simulink model "CtrlStrct_VNT_Level1_TW"  (R2018a)
settings: Solver=FixedStepAuto  StartTime=0.0  StopTime=10.0  FixedStep=0.001  RelTol=1e-3  EnableMultiTasking=on
PreLoadFcn:
  | CtrlStrct_SmplCAN_BusInfo
libraries: canmsglib x55, simulink x1
(part 3 of 3)

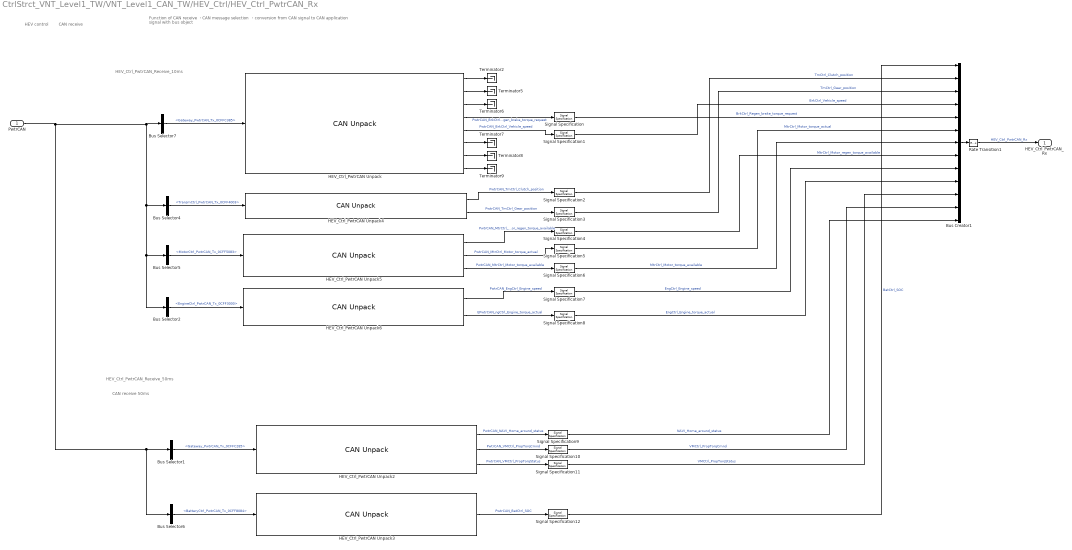
== system CtrlStrct_VNT_Level1_TW/VNT_Level1_CAN_TW/HEV_Ctrl/HEV_Ctrl_PwtrCAN_Rx ==
  note: HEV_Ctrl_PwtrCAN_Receive_50ms
  note: HEV_Ctrl_PwtrCAN_Receive_10ms
  note: CAN receive
  note: HEV control
  note: Function of CAN receive
      | ・CAN message selection
      | ・conversion from CAN signal to CAN application signal with bus object
  note: CAN receive 50ms
  PwtrCAN : Inport
  Bus Creator1 : BusCreator  Inputs=13  OutDataTypeStr=Bus: HEV_Ctrl_PwtrCAN_Rx_Bus
  Bus Selector1 : BusSelector  OutputSignals=Gateway_PwtrCAN_Tx_0CFFC285
  Bus Selector2 : BusSelector  OutputSignals=EngineCtrl_PwtrCAN_Tx_0CFF3000
  Bus Selector4 : BusSelector  OutputSignals=TransmCtrl_PwtrCAN_Tx_0CFF4003
  Bus Selector5 : BusSelector  OutputSignals=MotorCtrl_PwtrCAN_Tx_0CFF5083
  Bus Selector6 : BusSelector  OutputSignals=BatteryCtrl_PwtrCAN_Tx_0CFF8084
  Bus Selector7 : BusSelector  OutputSignals=Gateway_PwtrCAN_Tx_0CFFC385
  HEV_Ctrl_PwtrCAN Unpack : canmsglib/CAN Unpack  CANdbFile=HEV_CANDB.dbc  MsgList=Gateway_PwtrCAN_Tx_2  MsgName=Gateway_PwtrCAN_Tx_2  MsgIDType=Extended (29-bit identifier)  MsgIdentifier=218088325  MsgLength=8  SignalInfo=BdyCtrl_Door_open_flag_G$60$1$1$2$1$0$1$0$0$1$#BdyCtrl_Engine_hood_open_flg_G$59$1$1$2$1$0$1$0$0$1$#BdyCtrl_Idlestop_cancel_G$58$1$1$2$1$0$1$0$0$1$#BrkCtrl_Regen_brake_torque_re_G$16$16$1$1$1$0$1.000000e-02$0$-300$300$#BrkCtrl_Vehicle_speed_G$0$16$1$2$1$0$1.000000e-01$0$0$180$#HVAC_Ctrl_Idlestop_cancel_G$57$1$1$2$1$0$1$0$0$1$#HVAC_Ctrl_Idlestop_enbl_G$56$1$1$2$1$0$1$0$0$1$#StrgCtrl_Steer_angle_G$32$16$1$1$1$0$3.125000e-02$0$-720$720$#  NSignals=8  IDPort=off  TimestampPort=off  ErrorPort=off  RemotePort=off  LengthPort=off  StatusPort=off  StartBits=str2num('[int32(60);int32(59);int32(58);int32(16);int32(0);int32(57);int32(56);int32(32)]')  SignalSizes=str2num('[int32(1);int32(1);int32(1);int32(16);int32(16);int32(1);int32(1);int32(16)]')  ByteOrders=str2num('[int32(1);int32(1);int32(1);int32(1);int32(1);int32(1);int32(1);int32(1)]')  DataTypes=str2num('[int32(2);int32(2);int32(2);int32(1);int32(2);int32(2);int32(2);int32(1)]')  MultiplexTypes=str2num('[int32(1);int32(1);int32(1);int32(1);int32(1);int32(1);int32(1);int32(1)]')  MultiplexValues=str2num('[double(0);double(0);double(0);double(0);double(0);double(0);double(0);double(0)]')  Factors=str2num('[double(1);double(1);double(1);double(1.000000e-02);double(1.000000e-01);double(1);double(1);double(3.125000e-02)]')  Offsets=str2num('[double(0);double(0);double(0);double(0);double(0);double(0);double(0);double(0)]')  Minimums=str2num('[double(0);double(0);double(0);double(-300);double(0);double(0);double(0);double(-720)]')  Maximums=str2num('[double(1);double(1);double(1);double(300);double(180);double(1);double(1);double(720)]')  ApplyMinMax=off
      settings: AttributesFormatString=<CANdbFile = %<CANdbFile>>  SourceProductName=Simulink Real-Time  SourceProductBaseCode=XP  DataFormat=CANdb specified signals
  HEV_Ctrl_PwtrCAN Unpack2 : canmsglib/CAN Unpack  CANdbFile=HEV_CANDB.dbc  MsgList=Gateway_PwtrCAN_Tx_1  MsgName=Gateway_PwtrCAN_Tx_1  MsgIDType=Extended (29-bit identifier)  MsgIdentifier=218088069  MsgLength=8  SignalInfo=NAVI_Home_around_status_G$0$16$1$2$1$0$1$0$0$65535$#VMCtrl_PropTorqCmnd_G$24$16$1$1$1$0$1.000000e-02$0$-300$300$#VMCtrl_PropTorqStatus_G$16$8$1$2$1$0$1$0$0$7$#  NSignals=3  IDPort=off  TimestampPort=off  ErrorPort=off  RemotePort=off  LengthPort=off  StatusPort=off  StartBits=str2num('[int32(0);int32(24);int32(16)]')  SignalSizes=str2num('[int32(16);int32(16);int32(8)]')  ByteOrders=str2num('[int32(1);int32(1);int32(1)]')  DataTypes=str2num('[int32(2);int32(1);int32(2)]')  MultiplexTypes=str2num('[int32(1);int32(1);int32(1)]')  MultiplexValues=str2num('[double(0);double(0);double(0)]')  Factors=str2num('[double(1);double(1.000000e-02);double(1)]')  Offsets=str2num('[double(0);double(0);double(0)]')  Minimums=str2num('[double(0);double(-300);double(0)]')  Maximums=str2num('[double(65535);double(300);double(7)]')  ApplyMinMax=off
      settings: AttributesFormatString=<CANdbFile = %<CANdbFile>>  SourceProductName=Simulink Real-Time  SourceProductBaseCode=XP  DataFormat=CANdb specified signals
  HEV_Ctrl_PwtrCAN Unpack3 : canmsglib/CAN Unpack  CANdbFile=HEV_CANDB.dbc  MsgList=BatteryCtrl_PwtrCAN_Tx  MsgName=BatteryCtrl_PwtrCAN_Tx  MsgIDType=Extended (29-bit identifier)  MsgIdentifier=218071172  MsgLength=8  SignalInfo=BatCtrl_SOC$0$16$1$2$1$0$3.906250e-03$0$0$100$#  NSignals=1  IDPort=off  TimestampPort=off  ErrorPort=off  RemotePort=off  LengthPort=off  StatusPort=off  StartBits=str2num('[int32(0)]')  SignalSizes=str2num('[int32(16)]')  ByteOrders=str2num('[int32(1)]')  DataTypes=str2num('[int32(2)]')  MultiplexTypes=str2num('[int32(1)]')  MultiplexValues=str2num('[double(0)]')  Factors=str2num('[double(3.906250e-03)]')  Offsets=str2num('[double(0)]')  Minimums=str2num('[double(0)]')  Maximums=str2num('[double(100)]')  ApplyMinMax=off
      settings: AttributesFormatString=<CANdbFile = %<CANdbFile>>  SourceProductName=Simulink Real-Time  SourceProductBaseCode=XP  DataFormat=CANdb specified signals
  HEV_Ctrl_PwtrCAN Unpack4 : canmsglib/CAN Unpack  CANdbFile=HEV_CANDB.dbc  MsgList=TransmCtrl_PwtrCAN_Tx  MsgName=TransmCtrl_PwtrCAN_Tx  MsgIDType=Extended (29-bit identifier)  MsgIdentifier=218054659  MsgLength=8  SignalInfo=TmCtrl_Clutch_position$0$8$1$2$1$0$1.000000e-02$0$0$1$#TmCtrl_Gear_position$8$8$1$2$1$0$1$0$0$5$#  NSignals=2  IDPort=off  TimestampPort=off  ErrorPort=off  RemotePort=off  LengthPort=off  StatusPort=off  StartBits=str2num('[int32(0);int32(8)]')  SignalSizes=str2num('[int32(8);int32(8)]')  ByteOrders=str2num('[int32(1);int32(1)]')  DataTypes=str2num('[int32(2);int32(2)]')  MultiplexTypes=str2num('[int32(1);int32(1)]')  MultiplexValues=str2num('[double(0);double(0)]')  Factors=str2num('[double(1.000000e-02);double(1)]')  Offsets=str2num('[double(0);double(0)]')  Minimums=str2num('[double(0);double(0)]')  Maximums=str2num('[double(1);double(5)]')  ApplyMinMax=off
      settings: AttributesFormatString=<CANdbFile = %<CANdbFile>>  SourceProductName=Simulink Real-Time  SourceProductBaseCode=XP  DataFormat=CANdb specified signals
  HEV_Ctrl_PwtrCAN Unpack5 : canmsglib/CAN Unpack  CANdbFile=HEV_CANDB.dbc  MsgList=MotorCtrl_PwtrCAN_Tx  MsgName=MotorCtrl_PwtrCAN_Tx  MsgIDType=Extended (29-bit identifier)  MsgIdentifier=218058883  MsgLength=8  SignalInfo=MtrCtrl_Motor_regen_torque_avail$32$16$1$1$1$0$1.000000e-02$0$-300$300$#MtrCtrl_Motor_torque_actual$0$16$1$1$1$0$1.000000e-02$0$-300$300$#MtrCtrl_Motor_torque_available$16$16$1$1$1$0$1.000000e-02$0$-300$300$#  NSignals=3  IDPort=off  TimestampPort=off  ErrorPort=off  RemotePort=off  LengthPort=off  StatusPort=off  StartBits=str2num('[int32(32);int32(0);int32(16)]')  SignalSizes=str2num('[int32(16);int32(16);int32(16)]')  ByteOrders=str2num('[int32(1);int32(1);int32(1)]')  DataTypes=str2num('[int32(1);int32(1);int32(1)]')  MultiplexTypes=str2num('[int32(1);int32(1);int32(1)]')  MultiplexValues=str2num('[double(0);double(0);double(0)]')  Factors=str2num('[double(1.000000e-02);double(1.000000e-02);double(1.000000e-02)]')  Offsets=str2num('[double(0);double(0);double(0)]')  Minimums=str2num('[double(-300);double(-300);double(-300)]')  Maximums=str2num('[double(300);double(300);double(300)]')  ApplyMinMax=off
      settings: AttributesFormatString=<CANdbFile = %<CANdbFile>>  SourceProductName=Simulink Real-Time  SourceProductBaseCode=XP  DataFormat=CANdb specified signals
  HEV_Ctrl_PwtrCAN Unpack6 : canmsglib/CAN Unpack  CANdbFile=HEV_CANDB.dbc  MsgList=EngineCtrl_PwtrCAN_Tx  MsgName=EngineCtrl_PwtrCAN_Tx  MsgIDType=Extended (29-bit identifier)  MsgIdentifier=218050560  MsgLength=8  SignalInfo=EngCtrl_Engine_speed$0$16$1$2$1$0$1.250000e-01$0$0$8192$#EngCtrl_Engine_torque_actual$16$16$1$1$1$0$1.562500e-02$0$-300$300$#  NSignals=2  IDPort=off  TimestampPort=off  ErrorPort=off  RemotePort=off  LengthPort=off  StatusPort=off  StartBits=str2num('[int32(0);int32(16)]')  SignalSizes=str2num('[int32(16);int32(16)]')  ByteOrders=str2num('[int32(1);int32(1)]')  DataTypes=str2num('[int32(2);int32(1)]')  MultiplexTypes=str2num('[int32(1);int32(1)]')  MultiplexValues=str2num('[double(0);double(0)]')  Factors=str2num('[double(1.250000e-01);double(1.562500e-02)]')  Offsets=str2num('[double(0);double(0)]')  Minimums=str2num('[double(0);double(-300)]')  Maximums=str2num('[double(8192);double(300)]')  ApplyMinMax=off
      settings: AttributesFormatString=<CANdbFile = %<CANdbFile>>  SourceProductName=Simulink Real-Time  SourceProductBaseCode=XP  DataFormat=CANdb specified signals
  Rate Transition1 : RateTransition  Deterministic=off
      settings: AttributesFormatString=<Deterministic=%<Deterministic>>
  Signal Specification{,1..12} (13 alike) : SignalSpecification
  Terminator{2,5..9} (6 alike) : Terminator
  HEV_Ctrl_PwtrCAN_Rx : Outport
  wires:
  Rate Transition1/1 -> HEV_Ctrl_PwtrCAN_Rx/1  "HEV_Ctrl_PwtrCAN_Rx"
  Bus Creator1/1 -> Rate Transition1/1
  Signal Specification8/1 -> Bus Creator1/10  "EngCtrl_Engine_torque_actual"
  HEV_Ctrl_PwtrCAN Unpack/3 -> Terminator6/1
  HEV_Ctrl_PwtrCAN Unpack/6 -> Terminator7/1
  Signal Specification7/1 -> Bus Creator1/9  "EngCtrl_Engine_speed"
  HEV_Ctrl_PwtrCAN Unpack/1 -> Terminator2/1
  HEV_Ctrl_PwtrCAN Unpack/2 -> Terminator5/1
  HEV_Ctrl_PwtrCAN Unpack5/1 -> Signal Specification4/1  "PwtrCAN_MtrCtrl_Motor_regen_torque_available"
  Signal Specification6/1 -> Bus Creator1/7  "MtrCtrl_Motor_torque_available"
  HEV_Ctrl_PwtrCAN Unpack/5 -> Signal Specification1/1  "PwtrCAN_BrkCtrl_Vehicle_speed"
  HEV_Ctrl_PwtrCAN Unpack/4 -> Signal Specification/1  "PwtrCAN_BrkCtrl_Regen_brake_torque_request"
  HEV_Ctrl_PwtrCAN Unpack6/2 -> Signal Specification8/1  "EPwtrCAN_ngCtrl_Engine_torque_actual"
  Signal Specification2/1 -> Bus Creator1/2  "TmCtrl_Clutch_position"
  Signal Specification4/1 -> Bus Creator1/8  "MtrCtrl_Motor_regen_torque_available"
  HEV_Ctrl_PwtrCAN Unpack/8 -> Terminator9/1
  HEV_Ctrl_PwtrCAN Unpack5/2 -> Signal Specification5/1  "PwtrCAN_MtrCtrl_Motor_torque_actual"
  Signal Specification3/1 -> Bus Creator1/3  "TmCtrl_Gear_position"
  HEV_Ctrl_PwtrCAN Unpack4/1 -> Signal Specification2/1  "PwtrCAN_TmCtrl_Clutch_position"
  HEV_Ctrl_PwtrCAN Unpack6/1 -> Signal Specification7/1  "PwtrCAN_EngCtrl_Engine_speed"
  Signal Specification1/1 -> Bus Creator1/4  "BrkCtrl_Vehicle_speed"
  HEV_Ctrl_PwtrCAN Unpack4/2 -> Signal Specification3/1  "PwtrCAN_TmCtrl_Gear_position"
  HEV_Ctrl_PwtrCAN Unpack5/3 -> Signal Specification6/1  "PwtrCAN_MtrCtrl_Motor_torque_available"
  Signal Specification/1 -> Bus Creator1/5  "BrkCtrl_Regen_brake_torque_request"
  HEV_Ctrl_PwtrCAN Unpack/7 -> Terminator8/1
  Signal Specification5/1 -> Bus Creator1/6  "MtrCtrl_Motor_torque_actual"
  Bus Selector7/1 -> HEV_Ctrl_PwtrCAN Unpack/1  "<Gateway_PwtrCAN_Tx_0CFFC385>"
  Bus Selector5/1 -> HEV_Ctrl_PwtrCAN Unpack5/1  "<MotorCtrl_PwtrCAN_Tx_0CFF5083>"
  Bus Selector4/1 -> HEV_Ctrl_PwtrCAN Unpack4/1  "<TransmCtrl_PwtrCAN_Tx_0CFF4003>"
  Bus Selector2/1 -> HEV_Ctrl_PwtrCAN Unpack6/1  "<EngineCtrl_PwtrCAN_Tx_0CFF3000>"
  Signal Specification11/1 -> Bus Creator1/11  "VMCtrl_PropTorqStatus"
  Signal Specification12/1 -> Bus Creator1/1  "BatCtrl_SOC"
  HEV_Ctrl_PwtrCAN Unpack3/1 -> Signal Specification12/1  "PwtrCAN_BatCtrl_SOC"
  Signal Specification9/1 -> Bus Creator1/13  "NAVI_Home_around_status"
  Signal Specification10/1 -> Bus Creator1/12  "VMCtrl_PropTorqCmnd"
  HEV_Ctrl_PwtrCAN Unpack2/2 -> Signal Specification10/1  "PwtrCAN_VMCtrl_PropTorqCmnd"
  HEV_Ctrl_PwtrCAN Unpack2/3 -> Signal Specification11/1  "PwtrCAN_VMCtrl_PropTorqStatus"
  HEV_Ctrl_PwtrCAN Unpack2/1 -> Signal Specification9/1  "PwtrCAN_NAVI_Home_around_status"
  Bus Selector1/1 -> HEV_Ctrl_PwtrCAN Unpack2/1  "<Gateway_PwtrCAN_Tx_0CFFC285>"
  PwtrCAN/1 -> Bus Selector7/1, Bus Selector5/1, Bus Selector2/1, Bus Selector4/1, Bus Selector6/1, Bus Selector1/1
  Bus Selector6/1 -> HEV_Ctrl_PwtrCAN Unpack3/1  "<BatteryCtrl_PwtrCAN_Tx_0CFF8084>"

== system CtrlStrct_VNT_Level1_TW/VNT_Level1_CAN_TW/HVAC_Ctrl/HVAC_Ctrl_VehCAN Tx ==
  note: CAN transmit
  note: Function of CAN transmit
      | ・conversion fromCAN application signal to signal of CAN message
  note: HVAC Control
  HVAC_Ctrl_VehCAN_Tx_Apli : Inport
  Bus Creator1 : BusCreator  Inputs=1
  Bus Selector2 : BusSelector  OutputSignals=HVAC_Ctrl_Idlestop_cancel,HVAC_Ctrl_Idlestop_enbl
  HVAC_Ctrl_VehCAN Pack : canmsglib/CAN Pack  CANdbFile=HEV_CANDB.dbc  MsgList=HVAC_Ctrl_VehCAN_Tx  MsgName=HVAC_Ctrl_VehCAN_Tx  MsgIDType=Extended (29-bit identifier)  MsgIdentifier=218095751  MsgLength=8  SignalInfo=HVAC_Ctrl_Idlestop_cancel$1$1$1$2$1$0$1$0$0$1$#HVAC_Ctrl_Idlestop_enbl$0$1$1$2$1$0$1$0$0$1$#  NSignals=2  StartBits=str2num('[int32(1);int32(0)]')  SignalSizes=str2num('[int32(1);int32(1)]')  ByteOrders=str2num('[int32(1);int32(1)]')  DataTypes=str2num('[int32(2);int32(2)]')  MultiplexTypes=str2num('[int32(1);int32(1)]')  MultiplexValues=str2num('[double(0);double(0)]')  Factors=str2num('[double(1);double(1)]')  Offsets=str2num('[double(0);double(0)]')  Minimums=str2num('[double(0);double(0)]')  Maximums=str2num('[double(1);double(1)]')  Remote=off  ApplyMinMax=off  BusOutput=off
      settings: AttributesFormatString=<CANdbFile = %<CANdbFile>>  SourceProductName=Simulink Real-Time  SourceProductBaseCode=XP  DataFormat=CANdb specified signals
  HVAC_Ctrl_VehCAN_Tx : Outport
  wires:
  Bus Creator1/1 -> HVAC_Ctrl_VehCAN_Tx/1  "HVAC_Ctrl_VehCAN_Tx"
  HVAC_Ctrl_VehCAN_Tx_Apli/1 -> Bus Selector2/1
  HVAC_Ctrl_VehCAN Pack/1 -> Bus Creator1/1  "HVAC_Ctrl_VehCAN_Tx_0CFFE087"
  Bus Selector2/1 -> HVAC_Ctrl_VehCAN Pack/1  "<HVAC_Ctrl_Idlestop_cancel>"
  Bus Selector2/2 -> HVAC_Ctrl_VehCAN Pack/2  "<HVAC_Ctrl_Idlestop_enbl>"

== system CtrlStrct_VNT_Level1_TW/VNT_Level1_CAN_TW/HVAC_Ctrl/HVAC_Ctrl_VehCAN_Rx ==
  note: CAN receive
  note: Function of CAN receive
      | ・CAN message selection
      | ・conversion from CAN signal to CAN application signal with bus object
  note: HVAC Control
  VehCAN : Inport
  Bus Creator : BusCreator  Inputs=3
  HVAC_Ctrl_VehCAN_Receive_50ms : Subsystem
  Rate Transition1 : RateTransition  Deterministic=off
      settings: AttributesFormatString=<Deterministic=%<Deterministic>>
  HVAC_Ctrl_VehCAN_Rx : Outport
  wires:
  Rate Transition1/1 -> HVAC_Ctrl_VehCAN_Rx/1  "HVAC_Ctrl_VehCAN_Rx"
  VehCAN/1 -> HVAC_Ctrl_VehCAN_Receive_50ms/1(VehCAN_Msg)
  Bus Creator/1 -> Rate Transition1/1
  HVAC_Ctrl_VehCAN_Receive_50ms/1(EngCtrl_Engine_speed) -> Bus Creator/1
  HVAC_Ctrl_VehCAN_Receive_50ms/2(HEVCtrl_IdleStop_preparation_request) -> Bus Creator/2
  HVAC_Ctrl_VehCAN_Receive_50ms/3(HEVCtrl_IdleStop_status) -> Bus Creator/3

== system CtrlStrct_VNT_Level1_TW/VNT_Level1_CAN_TW/Motor_Ctrl/MotorCtrl_PwtrCAN Tx ==
  note: CAN transmit
  note: Motor Control
  note: Function of CAN transmit
      | ・conversion fromCAN application signal to signal of CAN message
  IMotorCtrl_PwtrCAN_Tx_Apli : Inport
  Bus Creator1 : BusCreator  Inputs=1
  Bus Selector1 : BusSelector  OutputSignals=MtrCtrl_Motor_regen_torque_available,MtrCtrl_Motor_torque_actual,MtrCtrl_Motor_torque_available
  MotorCtrl_PwtrCAN Pack : canmsglib/CAN Pack  CANdbFile=HEV_CANDB.dbc  MsgList=MotorCtrl_PwtrCAN_Tx  MsgName=MotorCtrl_PwtrCAN_Tx  MsgIDType=Extended (29-bit identifier)  MsgIdentifier=218058883  MsgLength=8  SignalInfo=MtrCtrl_Motor_regen_torque_avail$32$16$1$1$1$0$1.000000e-02$0$-300$300$#MtrCtrl_Motor_torque_actual$0$16$1$1$1$0$1.000000e-02$0$-300$300$#MtrCtrl_Motor_torque_available$16$16$1$1$1$0$1.000000e-02$0$-300$300$#  NSignals=3  StartBits=str2num('[int32(32);int32(0);int32(16)]')  SignalSizes=str2num('[int32(16);int32(16);int32(16)]')  ByteOrders=str2num('[int32(1);int32(1);int32(1)]')  DataTypes=str2num('[int32(1);int32(1);int32(1)]')  MultiplexTypes=str2num('[int32(1);int32(1);int32(1)]')  MultiplexValues=str2num('[double(0);double(0);double(0)]')  Factors=str2num('[double(1.000000e-02);double(1.000000e-02);double(1.000000e-02)]')  Offsets=str2num('[double(0);double(0);double(0)]')  Minimums=str2num('[double(-300);double(-300);double(-300)]')  Maximums=str2num('[double(300);double(300);double(300)]')  Remote=off  ApplyMinMax=off  BusOutput=off
      settings: AttributesFormatString=<CANdbFile = %<CANdbFile>>  SourceProductName=Simulink Real-Time  SourceProductBaseCode=XP  DataFormat=CANdb specified signals
  MotorCtrl_PwtrCAN_Tx_0CFF5083 : Outport
  wires:
  Bus Selector1/1 -> MotorCtrl_PwtrCAN Pack/1  "<MtrCtrl_Motor_regen_torque_available>"
  IMotorCtrl_PwtrCAN_Tx_Apli/1 -> Bus Selector1/1
  MotorCtrl_PwtrCAN Pack/1 -> Bus Creator1/1  "MotorCtrl_PwtrCAN_Tx_0CFF5083"
  Bus Selector1/3 -> MotorCtrl_PwtrCAN Pack/3  "<MtrCtrl_Motor_torque_available>"
  Bus Creator1/1 -> MotorCtrl_PwtrCAN_Tx_0CFF5083/1  "MotorCtrl_PwtrCAN_Tx"
  Bus Selector1/2 -> MotorCtrl_PwtrCAN Pack/2  "<MtrCtrl_Motor_torque_actual>"

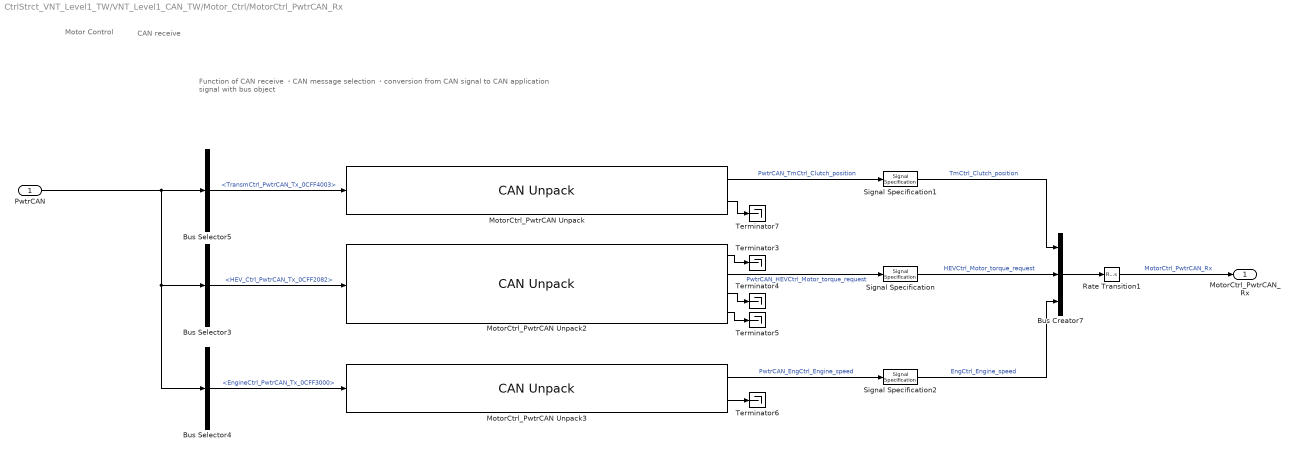
== system CtrlStrct_VNT_Level1_TW/VNT_Level1_CAN_TW/Motor_Ctrl/MotorCtrl_PwtrCAN_Rx ==
  note: CAN receive
  note: Motor Control
  note: Function of CAN receive
      | ・CAN message selection
      | ・conversion from CAN signal to CAN application signal with bus object
  PwtrCAN : Inport
  Bus Creator7 : BusCreator  Inputs=3
  Bus Selector3 : BusSelector  OutputSignals=HEV_Ctrl_PwtrCAN_Tx_0CFF2082
  Bus Selector4 : BusSelector  OutputSignals=EngineCtrl_PwtrCAN_Tx_0CFF3000
  Bus Selector5 : BusSelector  OutputSignals=TransmCtrl_PwtrCAN_Tx_0CFF4003
  MotorCtrl_PwtrCAN Unpack : canmsglib/CAN Unpack  CANdbFile=HEV_CANDB.dbc  MsgList=TransmCtrl_PwtrCAN_Tx  MsgName=TransmCtrl_PwtrCAN_Tx  MsgIDType=Extended (29-bit identifier)  MsgIdentifier=218054659  MsgLength=8  SignalInfo=TmCtrl_Clutch_position$0$8$1$2$1$0$1.000000e-02$0$0$1$#TmCtrl_Gear_position$8$8$1$2$1$0$1$0$0$5$#  NSignals=2  IDPort=off  TimestampPort=off  ErrorPort=off  RemotePort=off  LengthPort=off  StatusPort=off  StartBits=str2num('[int32(0);int32(8)]')  SignalSizes=str2num('[int32(8);int32(8)]')  ByteOrders=str2num('[int32(1);int32(1)]')  DataTypes=str2num('[int32(2);int32(2)]')  MultiplexTypes=str2num('[int32(1);int32(1)]')  MultiplexValues=str2num('[double(0);double(0)]')  Factors=str2num('[double(1.000000e-02);double(1)]')  Offsets=str2num('[double(0);double(0)]')  Minimums=str2num('[double(0);double(0)]')  Maximums=str2num('[double(1);double(5)]')  ApplyMinMax=off
      settings: AttributesFormatString=<CANdbFile = %<CANdbFile>>  SourceProductName=Simulink Real-Time  SourceProductBaseCode=XP  DataFormat=CANdb specified signals
  MotorCtrl_PwtrCAN Unpack2 : canmsglib/CAN Unpack  CANdbFile=HEV_CANDB.dbc  MsgList=HEV_Ctrl_PwtrCAN_Tx_1  MsgName=HEV_Ctrl_PwtrCAN_Tx_1  MsgIDType=Extended (29-bit identifier)  MsgIdentifier=218046594  MsgLength=8  SignalInfo=HEVCtrl_Engine_torque_request$0$16$1$1$1$0$1.562500e-02$0$-300$300$#HEVCtrl_Motor_torque_request$16$16$1$1$1$0$1.562500e-02$0$-300$300$#HEVCtrl_Regen_brake_torque_actua$48$16$1$1$1$0$6.250000e-02$0$-300$3000$#HEVCtrl_Regen_brake_torque_avail$32$16$1$1$1$0$6.250000e-02$0$-300$3000$#  NSignals=4  IDPort=off  TimestampPort=off  ErrorPort=off  RemotePort=off  LengthPort=off  StatusPort=off  StartBits=str2num('[int32(0);int32(16);int32(48);int32(32)]')  SignalSizes=str2num('[int32(16);int32(16);int32(16);int32(16)]')  ByteOrders=str2num('[int32(1);int32(1);int32(1);int32(1)]')  DataTypes=str2num('[int32(1);int32(1);int32(1);int32(1)]')  MultiplexTypes=str2num('[int32(1);int32(1);int32(1);int32(1)]')  MultiplexValues=str2num('[double(0);double(0);double(0);double(0)]')  Factors=str2num('[double(1.562500e-02);double(1.562500e-02);double(6.250000e-02);double(6.250000e-02)]')  Offsets=str2num('[double(0);double(0);double(0);double(0)]')  Minimums=str2num('[double(-300);double(-300);double(-300);double(-300)]')  Maximums=str2num('[double(300);double(300);double(3000);double(3000)]')  ApplyMinMax=off
      settings: AttributesFormatString=<CANdbFile = %<CANdbFile>>  SourceProductName=Simulink Real-Time  SourceProductBaseCode=XP  DataFormat=CANdb specified signals
  MotorCtrl_PwtrCAN Unpack3 : canmsglib/CAN Unpack  CANdbFile=HEV_CANDB.dbc  MsgList=EngineCtrl_PwtrCAN_Tx  MsgName=EngineCtrl_PwtrCAN_Tx  MsgIDType=Extended (29-bit identifier)  MsgIdentifier=218050560  MsgLength=8  SignalInfo=EngCtrl_Engine_speed$0$16$1$2$1$0$1.250000e-01$0$0$8192$#EngCtrl_Engine_torque_actual$16$16$1$1$1$0$1.562500e-02$0$-300$300$#  NSignals=2  IDPort=off  TimestampPort=off  ErrorPort=off  RemotePort=off  LengthPort=off  StatusPort=off  StartBits=str2num('[int32(0);int32(16)]')  SignalSizes=str2num('[int32(16);int32(16)]')  ByteOrders=str2num('[int32(1);int32(1)]')  DataTypes=str2num('[int32(2);int32(1)]')  MultiplexTypes=str2num('[int32(1);int32(1)]')  MultiplexValues=str2num('[double(0);double(0)]')  Factors=str2num('[double(1.250000e-01);double(1.562500e-02)]')  Offsets=str2num('[double(0);double(0)]')  Minimums=str2num('[double(0);double(-300)]')  Maximums=str2num('[double(8192);double(300)]')  ApplyMinMax=off
      settings: AttributesFormatString=<CANdbFile = %<CANdbFile>>  SourceProductName=Simulink Real-Time  SourceProductBaseCode=XP  DataFormat=CANdb specified signals
  Rate Transition1 : RateTransition  Deterministic=off
      settings: AttributesFormatString=<Deterministic=%<Deterministic>>
  Signal Specification : SignalSpecification
  Signal Specification1 : SignalSpecification
  Signal Specification2 : SignalSpecification
  Terminator{3..7} (5 alike) : Terminator
  MotorCtrl_PwtrCAN_Rx : Outport
  wires:
  Rate Transition1/1 -> MotorCtrl_PwtrCAN_Rx/1  "MotorCtrl_PwtrCAN_Rx"
  Bus Creator7/1 -> Rate Transition1/1
  PwtrCAN/1 -> Bus Selector4/1, Bus Selector3/1, Bus Selector5/1
  Bus Selector3/1 -> MotorCtrl_PwtrCAN Unpack2/1  "<HEV_Ctrl_PwtrCAN_Tx_0CFF2082>"
  Bus Selector5/1 -> MotorCtrl_PwtrCAN Unpack/1  "<TransmCtrl_PwtrCAN_Tx_0CFF4003>"
  Bus Selector4/1 -> MotorCtrl_PwtrCAN Unpack3/1  "<EngineCtrl_PwtrCAN_Tx_0CFF3000>"
  Signal Specification2/1 -> Bus Creator7/3  "EngCtrl_Engine_speed"
  Signal Specification1/1 -> Bus Creator7/1  "TmCtrl_Clutch_position"
  Signal Specification/1 -> Bus Creator7/2  "HEVCtrl_Motor_torque_request"
  MotorCtrl_PwtrCAN Unpack2/2 -> Signal Specification/1  "PwtrCAN_HEVCtrl_Motor_torque_request"
  MotorCtrl_PwtrCAN Unpack/1 -> Signal Specification1/1  "PwtrCAN_TmCtrl_Clutch_position"
  MotorCtrl_PwtrCAN Unpack3/1 -> Signal Specification2/1  "PwtrCAN_EngCtrl_Engine_speed"
  MotorCtrl_PwtrCAN Unpack/2 -> Terminator7/1
  MotorCtrl_PwtrCAN Unpack2/1 -> Terminator3/1
  MotorCtrl_PwtrCAN Unpack2/4 -> Terminator5/1
  MotorCtrl_PwtrCAN Unpack3/2 -> Terminator6/1
  MotorCtrl_PwtrCAN Unpack2/3 -> Terminator4/1

== system CtrlStrct_VNT_Level1_TW/VNT_Level1_CAN_TW/NAVI/NAVI_InfoCAN_Rx ==
  note: CAN receive
  note: Navigation
  InfoCAN : Inport
  Bus Creator : BusCreator  Inputs=1  OutDataTypeStr=Bus: NAVI_InfoCAN_Rx_Bus
      settings: AttributesFormatString=<%<OutDataTypeStr>>
  Bus Selector1 : BusSelector  OutputSignals=Gateway_InfoCAN_Tx_0CFFC485
  NAVI_InfoCAN Unpack : canmsglib/CAN Unpack  CANdbFile=HEV_CANDB.dbc  MsgList=Gateway_InfoCAN_Tx  MsgName=Gateway_InfoCAN_Tx  MsgIDType=Extended (29-bit identifier)  MsgIdentifier=218099848  MsgLength=8  SignalInfo=BrkCtrl_Vehicle_speed_G1$0$16$1$2$1$0$1.000000e-01$0$0$180$#  NSignals=1  IDPort=off  TimestampPort=off  ErrorPort=off  RemotePort=off  LengthPort=off  StatusPort=off  StartBits=str2num('[int32(0)]')  SignalSizes=str2num('[int32(16)]')  ByteOrders=str2num('[int32(1)]')  DataTypes=str2num('[int32(2)]')  MultiplexTypes=str2num('[int32(1)]')  MultiplexValues=str2num('[double(0)]')  Factors=str2num('[double(1.000000e-01)]')  Offsets=str2num('[double(0)]')  Minimums=str2num('[double(0)]')  Maximums=str2num('[double(180)]')  ApplyMinMax=off
      settings: AttributesFormatString=<CANdbFile = %<CANdbFile>>  SourceProductName=Simulink Real-Time  SourceProductBaseCode=XP  DataFormat=CANdb specified signals
  Rate Transition1 : RateTransition  Deterministic=off
      settings: AttributesFormatString=<Deterministic=%<Deterministic>>
  Signal Specification : SignalSpecification
  NAVI_InfoCAN_Rx : Outport
  wires:
  Rate Transition1/1 -> NAVI_InfoCAN_Rx/1  "NAVI_InfoCAN_Rx"
  Bus Selector1/1 -> NAVI_InfoCAN Unpack/1  "<Gateway_InfoCAN_Tx_0CFFC485>"
  Bus Creator/1 -> Rate Transition1/1
  InfoCAN/1 -> Bus Selector1/1
  Signal Specification/1 -> Bus Creator/1  "BrkCtrl_Vehicle_speed"
  NAVI_InfoCAN Unpack/1 -> Signal Specification/1  "InfoCAN_BrkCtrl_Vehicle_speed"

== system CtrlStrct_VNT_Level1_TW/VNT_Level1_CAN_TW/NAVI/NAVI_InfoCAN_Tx ==
  note: CAN transmit
  note: Navigation
  NAVI_InfoCAN_Tx_Apli : Inport
  Bus Creator1 : BusCreator  Inputs=1
  Bus Selector3 : BusSelector  OutputSignals=NAVI_Home_around_status,NAVI_Road_information
  NAVI_InfoCAN Pack : canmsglib/CAN Pack  CANdbFile=HEV_CANDB.dbc  MsgList=NAVI_InfoCAN_Tx  MsgName=NAVI_InfoCAN_Tx  MsgIDType=Extended (29-bit identifier)  MsgIdentifier=218083356  MsgLength=8  SignalInfo=NAVI_Home_around_status$16$16$1$2$1$0$1$0$0$65535$#NAVI_Road_information$0$16$1$2$1$0$1$0$0$65535$#  NSignals=2  StartBits=str2num('[int32(16);int32(0)]')  SignalSizes=str2num('[int32(16);int32(16)]')  ByteOrders=str2num('[int32(1);int32(1)]')  DataTypes=str2num('[int32(2);int32(2)]')  MultiplexTypes=str2num('[int32(1);int32(1)]')  MultiplexValues=str2num('[double(0);double(0)]')  Factors=str2num('[double(1);double(1)]')  Offsets=str2num('[double(0);double(0)]')  Minimums=str2num('[double(0);double(0)]')  Maximums=str2num('[double(65535);double(65535)]')  Remote=off  ApplyMinMax=off  BusOutput=off
      settings: AttributesFormatString=<CANdbFile = %<CANdbFile>>  SourceProductName=Simulink Real-Time  SourceProductBaseCode=XP  DataFormat=CANdb specified signals
  NAVI_InfoCAN_Tx : Outport
  wires:
  Bus Creator1/1 -> NAVI_InfoCAN_Tx/1  "NAVI_InfoCAN_Tx"
  Bus Selector3/1 -> NAVI_InfoCAN Pack/1  "<NAVI_Home_around_status>"
  NAVI_InfoCAN Pack/1 -> Bus Creator1/1  "NAVI_InfoCAN_Tx_0CFFB01C"
  Bus Selector3/2 -> NAVI_InfoCAN Pack/2  "<NAVI_Road_information>"
  NAVI_InfoCAN_Tx_Apli/1 -> Bus Selector3/1

== system CtrlStrct_VNT_Level1_TW/VNT_Level1_CAN_TW/Radar/Radar_InfoCAN_Rx ==
  note: Radar Detection
  note: CAN receive
  note: Function of CAN receive
      | ・CAN message selection
      | ・conversion from CAN signal to CAN application signal with bus object
  InfoCAN : Inport
  Bus Creator : BusCreator  Inputs=1
  Bus Selector1 : BusSelector  OutputSignals=Gateway_InfoCAN_Tx_0CFFC485
  Radar_InfoCAN Unpack : canmsglib/CAN Unpack  CANdbFile=HEV_CANDB.dbc  MsgList=Gateway_InfoCAN_Tx  MsgName=Gateway_InfoCAN_Tx  MsgIDType=Extended (29-bit identifier)  MsgIdentifier=218099848  MsgLength=8  SignalInfo=BrkCtrl_Vehicle_speed_G1$0$16$1$2$1$0$1.000000e-01$0$0$180$#  NSignals=1  IDPort=off  TimestampPort=off  ErrorPort=off  RemotePort=off  LengthPort=off  StatusPort=off  StartBits=str2num('[int32(0)]')  SignalSizes=str2num('[int32(16)]')  ByteOrders=str2num('[int32(1)]')  DataTypes=str2num('[int32(2)]')  MultiplexTypes=str2num('[int32(1)]')  MultiplexValues=str2num('[double(0)]')  Factors=str2num('[double(1.000000e-01)]')  Offsets=str2num('[double(0)]')  Minimums=str2num('[double(0)]')  Maximums=str2num('[double(180)]')  ApplyMinMax=off
      settings: AttributesFormatString=<CANdbFile = %<CANdbFile>>  SourceProductName=Simulink Real-Time  SourceProductBaseCode=XP  DataFormat=CANdb specified signals
  Rate Transition1 : RateTransition  Deterministic=off
      settings: AttributesFormatString=<Deterministic=%<Deterministic>>
  Signal Specification : SignalSpecification
  Radar_InfoCAN_Rx : Outport
  wires:
  Rate Transition1/1 -> Radar_InfoCAN_Rx/1  "Radar_InfoCAN_Rx"
  Bus Selector1/1 -> Radar_InfoCAN Unpack/1  "<Gateway_InfoCAN_Tx_0CFFC485>"
  Bus Creator/1 -> Rate Transition1/1
  InfoCAN/1 -> Bus Selector1/1
  Signal Specification/1 -> Bus Creator/1  "BrkCtrl_Vehicle_speed"
  Radar_InfoCAN Unpack/1 -> Signal Specification/1  "InfoCAN_BrkCtrl_Vehicle_speed"

== system CtrlStrct_VNT_Level1_TW/VNT_Level1_CAN_TW/Radar/Radar_InfoCAN_Tx ==
  note: Radar Detection
  note: CAN transmit
  note: Function of CAN transmit
      | ・conversion fromCAN application signal to signal of CAN message
  Radar_InfoCAN_Tx_Apli : Inport
  Bus Creator1 : BusCreator  Inputs=1
  Bus Selector3 : BusSelector  OutputSignals=Radar_Relative_distance,Radar_Relative_velocity
  Radar_InfoCAN Pack : canmsglib/CAN Pack  CANdbFile=HEV_CANDB.dbc  MsgList=Radar_InfoCAN_Tx  MsgName=Radar_InfoCAN_Tx  MsgIDType=Extended (29-bit identifier)  MsgIdentifier=218038400  MsgLength=8  SignalInfo=Radar_Relative_distance$0$16$1$2$1$0$1.000000e-02$0$0$500$#Radar_Relative_velocity$16$16$1$1$1$0$1.000000e-02$0$-50$50$#  NSignals=2  StartBits=str2num('[int32(0);int32(16)]')  SignalSizes=str2num('[int32(16);int32(16)]')  ByteOrders=str2num('[int32(1);int32(1)]')  DataTypes=str2num('[int32(2);int32(1)]')  MultiplexTypes=str2num('[int32(1);int32(1)]')  MultiplexValues=str2num('[double(0);double(0)]')  Factors=str2num('[double(1.000000e-02);double(1.000000e-02)]')  Offsets=str2num('[double(0);double(0)]')  Minimums=str2num('[double(0);double(-50)]')  Maximums=str2num('[double(500);double(50)]')  Remote=off  ApplyMinMax=off  BusOutput=off
      settings: AttributesFormatString=<CANdbFile = %<CANdbFile>>  SourceProductName=Simulink Real-Time  SourceProductBaseCode=XP  DataFormat=CANdb specified signals
  Radar_InfoCAN_Tx : Outport
  wires:
  Bus Creator1/1 -> Radar_InfoCAN_Tx/1  "Radar_InfoCAN_Tx"
  Radar_InfoCAN_Tx_Apli/1 -> Bus Selector3/1
  Radar_InfoCAN Pack/1 -> Bus Creator1/1  "Radar_InfoCAN_Tx_0CFF0080"
  Bus Selector3/2 -> Radar_InfoCAN Pack/2  "<Radar_Relative_velocity>"
  Bus Selector3/1 -> Radar_InfoCAN Pack/1  "<Radar_Relative_distance>"

== system CtrlStrct_VNT_Level1_TW/VNT_Level1_CAN_TW/Steer_Ctrl/SteerCtrl_VehCAN Tx ==
  note: CAN transmit
  note: Function of CAN transmit
      | ・conversion fromCAN application signal to signal of CAN message
  note: Steering Control
  SteerCtrl_VehCAN_Tx_Apli : Inport
  Bus Creator1 : BusCreator  Inputs=1
  Bus Selector1 : BusSelector  OutputSignals=StrgCtrl_Steer_angle
  SteerCtrl_VehCAN Pack : canmsglib/CAN Pack  CANdbFile=HEV_CANDB.dbc  MsgList=SteerCtrl_VehCAN_Tx  MsgName=SteerCtrl_VehCAN_Tx  MsgIDType=Extended (29-bit identifier)  MsgIdentifier=218066963  MsgLength=8  SignalInfo=StrgCtrl_Steer_angle$0$16$1$1$1$0$3.125000e-02$0$-720$720$#  NSignals=1  StartBits=str2num('[int32(0)]')  SignalSizes=str2num('[int32(16)]')  ByteOrders=str2num('[int32(1)]')  DataTypes=str2num('[int32(1)]')  MultiplexTypes=str2num('[int32(1)]')  MultiplexValues=str2num('[double(0)]')  Factors=str2num('[double(3.125000e-02)]')  Offsets=str2num('[double(0)]')  Minimums=str2num('[double(-720)]')  Maximums=str2num('[double(720)]')  Remote=off  ApplyMinMax=off  BusOutput=off
      settings: AttributesFormatString=<CANdbFile = %<CANdbFile>>  SourceProductName=Simulink Real-Time  SourceProductBaseCode=XP  DataFormat=CANdb specified signals
  SteerCtrl_VehCAN_Tx : Outport
  wires:
  Bus Creator1/1 -> SteerCtrl_VehCAN_Tx/1  "SteerCtrl_VehCAN_Tx"
  SteerCtrl_VehCAN_Tx_Apli/1 -> Bus Selector1/1
  Bus Selector1/1 -> SteerCtrl_VehCAN Pack/1  "<StrgCtrl_Steer_angle>"
  SteerCtrl_VehCAN Pack/1 -> Bus Creator1/1  "SteerCtrl_VehCAN_Tx_0CFF7013"

== system CtrlStrct_VNT_Level1_TW/VNT_Level1_CAN_TW/Steer_Ctrl/SteerCtrl_VehCAN_Rx ==
  note: CAN receive
  note: Function of CAN receive
      | ・CAN message selection
      | ・conversion from CAN signal to CAN application signal with bus object
  note: Steering Control
  VehCAN : Inport
  Bus Creator : BusCreator  Inputs=1
  Bus Selector7 : BusSelector  OutputSignals=BrakeCtrl_VehCAN_Tx_0CFF600B
  Rate Transition1 : RateTransition  Deterministic=off
      settings: AttributesFormatString=<Deterministic=%<Deterministic>>
  Signal Specification : SignalSpecification
  SteerCtrl_VehCAN Unpack : canmsglib/CAN Unpack  CANdbFile=HEV_CANDB.dbc  MsgList=BrakeCtrl_VehCAN_Tx  MsgName=BrakeCtrl_VehCAN_Tx  MsgIDType=Extended (29-bit identifier)  MsgIdentifier=218062859  MsgLength=8  SignalInfo=BrkCtrl_Regen_brake_torque_reque$16$16$1$1$1$0$1.000000e-02$0$-300$300$#BrkCtrl_Vehicle_speed$0$16$1$2$1$0$1.000000e-01$0$0$180$#  NSignals=2  IDPort=off  TimestampPort=off  ErrorPort=off  RemotePort=off  LengthPort=off  StatusPort=off  StartBits=str2num('[int32(16);int32(0)]')  SignalSizes=str2num('[int32(16);int32(16)]')  ByteOrders=str2num('[int32(1);int32(1)]')  DataTypes=str2num('[int32(1);int32(2)]')  MultiplexTypes=str2num('[int32(1);int32(1)]')  MultiplexValues=str2num('[double(0);double(0)]')  Factors=str2num('[double(1.000000e-02);double(1.000000e-01)]')  Offsets=str2num('[double(0);double(0)]')  Minimums=str2num('[double(-300);double(0)]')  Maximums=str2num('[double(300);double(180)]')  ApplyMinMax=off
      settings: AttributesFormatString=<CANdbFile = %<CANdbFile>>  SourceProductName=Simulink Real-Time  SourceProductBaseCode=XP  DataFormat=CANdb specified signals
  Terminator4 : Terminator
  SteerCtrl_VehCAN_Rx : Outport
  wires:
  Rate Transition1/1 -> SteerCtrl_VehCAN_Rx/1  "SteerCtrl_VehCAN_Rx"
  Bus Selector7/1 -> SteerCtrl_VehCAN Unpack/1  "<BrakeCtrl_VehCAN_Tx_0CFF600B>"
  Bus Creator/1 -> Rate Transition1/1
  VehCAN/1 -> Bus Selector7/1
  SteerCtrl_VehCAN Unpack/2 -> Signal Specification/1  "VehCAN_BrkCtrl_Vehicle_speed"
  Signal Specification/1 -> Bus Creator/1  "BrkCtrl_Vehicle_speed"
  SteerCtrl_VehCAN Unpack/1 -> Terminator4/1  "VehCAN_BrkCtrl_Regen_brake_torque_request"

== system CtrlStrct_VNT_Level1_TW/VNT_Level1_CAN_TW/Transms_Ctrl/TransmCtrl_PwtrCAN Tx ==
  note: CAN transmit
  note: Transmission Control
  note: Function of CAN transmit
      | ・conversion fromCAN application signal to signal of CAN message
  TransmCtrl_PwtrCAN_Tx_Apli : Inport
  Bus Creator1 : BusCreator  Inputs=1
  Bus Selector2 : BusSelector  OutputSignals=TmCtrl_Clutch_position,TmCtrl_Gear_position
  TransmCtrl_PwtrCAN Pack : canmsglib/CAN Pack  CANdbFile=HEV_CANDB.dbc  MsgList=TransmCtrl_PwtrCAN_Tx  MsgName=TransmCtrl_PwtrCAN_Tx  MsgIDType=Extended (29-bit identifier)  MsgIdentifier=218054659  MsgLength=8  SignalInfo=TmCtrl_Clutch_position$0$8$1$2$1$0$1.000000e-02$0$0$1$#TmCtrl_Gear_position$8$8$1$2$1$0$1$0$0$5$#  NSignals=2  StartBits=str2num('[int32(0);int32(8)]')  SignalSizes=str2num('[int32(8);int32(8)]')  ByteOrders=str2num('[int32(1);int32(1)]')  DataTypes=str2num('[int32(2);int32(2)]')  MultiplexTypes=str2num('[int32(1);int32(1)]')  MultiplexValues=str2num('[double(0);double(0)]')  Factors=str2num('[double(1.000000e-02);double(1)]')  Offsets=str2num('[double(0);double(0)]')  Minimums=str2num('[double(0);double(0)]')  Maximums=str2num('[double(1);double(5)]')  Remote=off  ApplyMinMax=off  BusOutput=off
      settings: AttributesFormatString=<CANdbFile = %<CANdbFile>>  SourceProductName=Simulink Real-Time  SourceProductBaseCode=XP  DataFormat=CANdb specified signals
  TransmCtrl_PwtrCAN_Tx : Outport
  wires:
  Bus Selector2/1 -> TransmCtrl_PwtrCAN Pack/1  "<TmCtrl_Clutch_position>"
  Bus Selector2/2 -> TransmCtrl_PwtrCAN Pack/2  "<TmCtrl_Gear_position>"
  Bus Creator1/1 -> TransmCtrl_PwtrCAN_Tx/1  "TransmCtrl_PwtrCAN_Tx"
  TransmCtrl_PwtrCAN Pack/1 -> Bus Creator1/1  "TransmCtrl_PwtrCAN_Tx_0CFF4003"
  TransmCtrl_PwtrCAN_Tx_Apli/1 -> Bus Selector2/1

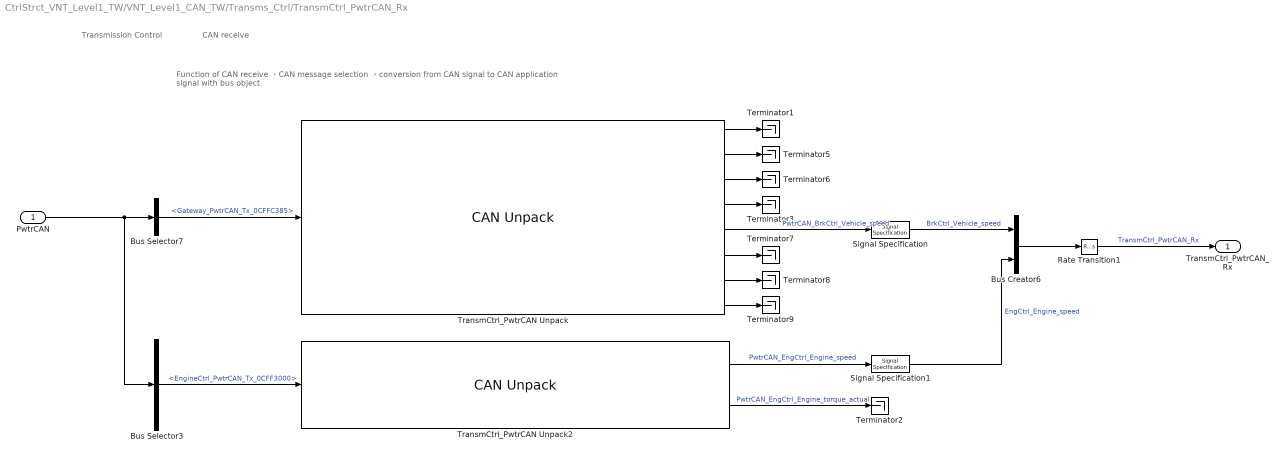
== system CtrlStrct_VNT_Level1_TW/VNT_Level1_CAN_TW/Transms_Ctrl/TransmCtrl_PwtrCAN_Rx ==
  note: CAN receive
  note: Function of CAN receive
      | ・CAN message selection
      | ・conversion from CAN signal to CAN application signal with bus object
  note: Transmission Control
  PwtrCAN : Inport
  Bus Creator6 : BusCreator  Inputs=2
  Bus Selector3 : BusSelector  OutputSignals=EngineCtrl_PwtrCAN_Tx_0CFF3000
  Bus Selector7 : BusSelector  OutputSignals=Gateway_PwtrCAN_Tx_0CFFC385
  Rate Transition1 : RateTransition  Deterministic=off
      settings: AttributesFormatString=<Deterministic=%<Deterministic>>
  Signal Specification : SignalSpecification
  Signal Specification1 : SignalSpecification
  Terminator{1..3,5..9} (8 alike) : Terminator
  TransmCtrl_PwtrCAN Unpack : canmsglib/CAN Unpack  CANdbFile=HEV_CANDB.dbc  MsgList=Gateway_PwtrCAN_Tx_2  MsgName=Gateway_PwtrCAN_Tx_2  MsgIDType=Extended (29-bit identifier)  MsgIdentifier=218088325  MsgLength=8  SignalInfo=BdyCtrl_Door_open_flag_G$60$1$1$2$1$0$1$0$0$1$#BdyCtrl_Engine_hood_open_flg_G$59$1$1$2$1$0$1$0$0$1$#BdyCtrl_Idlestop_cancel_G$58$1$1$2$1$0$1$0$0$1$#BrkCtrl_Regen_brake_torque_re_G$16$16$1$1$1$0$1.000000e-02$0$-300$300$#BrkCtrl_Vehicle_speed_G$0$16$1$2$1$0$1.000000e-01$0$0$180$#HVAC_Ctrl_Idlestop_cancel_G$57$1$1$2$1$0$1$0$0$1$#HVAC_Ctrl_Idlestop_enbl_G$56$1$1$2$1$0$1$0$0$1$#StrgCtrl_Steer_angle_G$32$16$1$1$1$0$3.125000e-02$0$-720$720$#  NSignals=8  IDPort=off  TimestampPort=off  ErrorPort=off  RemotePort=off  LengthPort=off  StatusPort=off  StartBits=str2num('[int32(60);int32(59);int32(58);int32(16);int32(0);int32(57);int32(56);int32(32)]')  SignalSizes=str2num('[int32(1);int32(1);int32(1);int32(16);int32(16);int32(1);int32(1);int32(16)]')  ByteOrders=str2num('[int32(1);int32(1);int32(1);int32(1);int32(1);int32(1);int32(1);int32(1)]')  DataTypes=str2num('[int32(2);int32(2);int32(2);int32(1);int32(2);int32(2);int32(2);int32(1)]')  MultiplexTypes=str2num('[int32(1);int32(1);int32(1);int32(1);int32(1);int32(1);int32(1);int32(1)]')  MultiplexValues=str2num('[double(0);double(0);double(0);double(0);double(0);double(0);double(0);double(0)]')  Factors=str2num('[double(1);double(1);double(1);double(1.000000e-02);double(1.000000e-01);double(1);double(1);double(3.125000e-02)]')  Offsets=str2num('[double(0);double(0);double(0);double(0);double(0);double(0);double(0);double(0)]')  Minimums=str2num('[double(0);double(0);double(0);double(-300);double(0);double(0);double(0);double(-720)]')  Maximums=str2num('[double(1);double(1);double(1);double(300);double(180);double(1);double(1);double(720)]')  ApplyMinMax=off
      settings: AttributesFormatString=<CANdbFile = %<CANdbFile>>  SourceProductName=Simulink Real-Time  SourceProductBaseCode=XP  DataFormat=CANdb specified signals
  TransmCtrl_PwtrCAN Unpack2 : canmsglib/CAN Unpack  CANdbFile=HEV_CANDB.dbc  MsgList=EngineCtrl_PwtrCAN_Tx  MsgName=EngineCtrl_PwtrCAN_Tx  MsgIDType=Extended (29-bit identifier)  MsgIdentifier=218050560  MsgLength=8  SignalInfo=EngCtrl_Engine_speed$0$16$1$2$1$0$1.250000e-01$0$0$8192$#EngCtrl_Engine_torque_actual$16$16$1$1$1$0$1.562500e-02$0$-300$300$#  NSignals=2  IDPort=off  TimestampPort=off  ErrorPort=off  RemotePort=off  LengthPort=off  StatusPort=off  StartBits=str2num('[int32(0);int32(16)]')  SignalSizes=str2num('[int32(16);int32(16)]')  ByteOrders=str2num('[int32(1);int32(1)]')  DataTypes=str2num('[int32(2);int32(1)]')  MultiplexTypes=str2num('[int32(1);int32(1)]')  MultiplexValues=str2num('[double(0);double(0)]')  Factors=str2num('[double(1.250000e-01);double(1.562500e-02)]')  Offsets=str2num('[double(0);double(0)]')  Minimums=str2num('[double(0);double(-300)]')  Maximums=str2num('[double(8192);double(300)]')  ApplyMinMax=off
      settings: AttributesFormatString=<CANdbFile = %<CANdbFile>>  SourceProductName=Simulink Real-Time  SourceProductBaseCode=XP  DataFormat=CANdb specified signals
  TransmCtrl_PwtrCAN_Rx : Outport
  wires:
  Bus Creator6/1 -> Rate Transition1/1
  Rate Transition1/1 -> TransmCtrl_PwtrCAN_Rx/1  "TransmCtrl_PwtrCAN_Rx"
  PwtrCAN/1 -> Bus Selector3/1, Bus Selector7/1
  Bus Selector7/1 -> TransmCtrl_PwtrCAN Unpack/1  "<Gateway_PwtrCAN_Tx_0CFFC385>"
  Bus Selector3/1 -> TransmCtrl_PwtrCAN Unpack2/1  "<EngineCtrl_PwtrCAN_Tx_0CFF3000>"
  Signal Specification1/1 -> Bus Creator6/2  "EngCtrl_Engine_speed"
  Signal Specification/1 -> Bus Creator6/1  "BrkCtrl_Vehicle_speed"
  TransmCtrl_PwtrCAN Unpack2/1 -> Signal Specification1/1  "PwtrCAN_EngCtrl_Engine_speed"
  TransmCtrl_PwtrCAN Unpack/5 -> Signal Specification/1  "PwtrCAN_BrkCtrl_Vehicle_speed"
  TransmCtrl_PwtrCAN Unpack2/2 -> Terminator2/1  "PwtrCAN_EngCtrl_Engine_torque_actual"
  TransmCtrl_PwtrCAN Unpack/1 -> Terminator1/1
  TransmCtrl_PwtrCAN Unpack/3 -> Terminator6/1
  TransmCtrl_PwtrCAN Unpack/6 -> Terminator7/1
  TransmCtrl_PwtrCAN Unpack/7 -> Terminator8/1
  TransmCtrl_PwtrCAN Unpack/4 -> Terminator3/1
  TransmCtrl_PwtrCAN Unpack/8 -> Terminator9/1
  TransmCtrl_PwtrCAN Unpack/2 -> Terminator5/1

== system CtrlStrct_VNT_Level1_TW/VNT_Level1_CAN_TW/VM_Ctrl/VM_Ctrl_VehCAN Tx ==
  note: CAN transmit
  note: Function of CAN transmit
      | ・conversion fromCAN application signal to signal of CAN message
  note: Vehicle Motion Control
  VM_Ctrl_VehCAN_Tx_Apli : Inport
  Bus Creator1 : BusCreator  Inputs=1
  Bus Selector3 : BusSelector  OutputSignals=VMCtrl_BrakeForceCmnd,VMCtrl_BrakeForceStatus,VMCtrl_PropTorqCmnd,VMCtrl_PropTorqStatus
  VM_Ctrl_VehCAN Pack : canmsglib/CAN Pack  CANdbFile=HEV_CANDB.dbc  MsgList=VM_Ctrl_VehCAN_Tx  MsgName=VM_Ctrl_VehCAN_Tx  MsgIDType=Extended (29-bit identifier)  MsgIdentifier=218091654  MsgLength=8  SignalInfo=VMCtrl_BrakeTorqCmnd$32$16$1$1$1$0$1.000000e-02$0$-300$300$#VMCtrl_BrakeTorqStatus$24$8$1$2$1$0$1$0$0$7$#VMCtrl_PropTorqCmnd$8$16$1$1$1$0$1.000000e-02$0$-300$300$#VMCtrl_PropTorqStatus$0$8$1$2$1$0$1$0$-Inf$Inf$#  NSignals=4  StartBits=str2num('[int32(32);int32(24);int32(8);int32(0)]')  SignalSizes=str2num('[int32(16);int32(8);int32(16);int32(8)]')  ByteOrders=str2num('[int32(1);int32(1);int32(1);int32(1)]')  DataTypes=str2num('[int32(1);int32(2);int32(1);int32(2)]')  MultiplexTypes=str2num('[int32(1);int32(1);int32(1);int32(1)]')  MultiplexValues=str2num('[double(0);double(0);double(0);double(0)]')  Factors=str2num('[double(1.000000e-02);double(1);double(1.000000e-02);double(1)]')  Offsets=str2num('[double(0);double(0);double(0);double(0)]')  Minimums=str2num('[double(-300);double(0);double(-300);double(-Inf)]')  Maximums=str2num('[double(300);double(7);double(300);double(Inf)]')  Remote=off  ApplyMinMax=off  BusOutput=off
      settings: AttributesFormatString=<CANdbFile = %<CANdbFile>>  SourceProductName=Simulink Real-Time  SourceProductBaseCode=XP  DataFormat=CANdb specified signals
  VM_Ctrl_VehCAN_Tx : Outport
  wires:
  Bus Selector3/4 -> VM_Ctrl_VehCAN Pack/4  "<VMCtrl_PropTorqStatus>"
  Bus Creator1/1 -> VM_Ctrl_VehCAN_Tx/1  "VM_Ctrl_VehCAN_Tx"
  VM_Ctrl_VehCAN_Tx_Apli/1 -> Bus Selector3/1
  VM_Ctrl_VehCAN Pack/1 -> Bus Creator1/1  "VM_Ctrl_VehCAN_Tx_0CFFD086"
  Bus Selector3/3 -> VM_Ctrl_VehCAN Pack/3  "<VMCtrl_PropTorqCmnd>"
  Bus Selector3/2 -> VM_Ctrl_VehCAN Pack/2  "<VMCtrl_BrakeForceStatus>"
  Bus Selector3/1 -> VM_Ctrl_VehCAN Pack/1  "<VMCtrl_BrakeForceCmnd>"

== system CtrlStrct_VNT_Level1_TW/VNT_Level1_CAN_TW/VM_Ctrl/VM_Ctrl_VehCAN_Rx ==
  note: CAN receive
  note: Function of CAN receive
      | ・CAN message selection
      | ・conversion from CAN signal to CAN application signal with bus object
  note: Vehicle Motion Control
  VehCAN : Inport
  Bus Creator : BusCreator  Inputs=1
  Bus Selector7 : BusSelector  OutputSignals=BrakeCtrl_VehCAN_Tx_0CFF600B
  Rate Transition1 : RateTransition  Deterministic=off
      settings: AttributesFormatString=<Deterministic=%<Deterministic>>
  Signal Specification : SignalSpecification
  Terminator4 : Terminator
  VM_Ctrl_VehCAN Unpack : canmsglib/CAN Unpack  CANdbFile=HEV_CANDB.dbc  MsgList=BrakeCtrl_VehCAN_Tx  MsgName=BrakeCtrl_VehCAN_Tx  MsgIDType=Extended (29-bit identifier)  MsgIdentifier=218062859  MsgLength=8  SignalInfo=BrkCtrl_Regen_brake_torque_reque$16$16$1$1$1$0$1.000000e-02$0$-300$300$#BrkCtrl_Vehicle_speed$0$16$1$2$1$0$1.000000e-01$0$0$180$#  NSignals=2  IDPort=off  TimestampPort=off  ErrorPort=off  RemotePort=off  LengthPort=off  StatusPort=off  StartBits=str2num('[int32(16);int32(0)]')  SignalSizes=str2num('[int32(16);int32(16)]')  ByteOrders=str2num('[int32(1);int32(1)]')  DataTypes=str2num('[int32(1);int32(2)]')  MultiplexTypes=str2num('[int32(1);int32(1)]')  MultiplexValues=str2num('[double(0);double(0)]')  Factors=str2num('[double(1.000000e-02);double(1.000000e-01)]')  Offsets=str2num('[double(0);double(0)]')  Minimums=str2num('[double(-300);double(0)]')  Maximums=str2num('[double(300);double(180)]')  ApplyMinMax=off
      settings: AttributesFormatString=<CANdbFile = %<CANdbFile>>  SourceProductName=Simulink Real-Time  SourceProductBaseCode=XP  DataFormat=CANdb specified signals
  VM_Ctrl_VehCAN_Rx : Outport
  wires:
  VehCAN/1 -> Bus Selector7/1
  Rate Transition1/1 -> VM_Ctrl_VehCAN_Rx/1  "VM_Ctrl_VehCAN_Rx"
  Bus Selector7/1 -> VM_Ctrl_VehCAN Unpack/1  "<BrakeCtrl_VehCAN_Tx_0CFF600B>"
  Bus Creator/1 -> Rate Transition1/1
  VM_Ctrl_VehCAN Unpack/2 -> Signal Specification/1  "VehCAN_BrkCtrl_Vehicle_speed"
  VM_Ctrl_VehCAN Unpack/1 -> Terminator4/1  "VehCAN_BrkCtrl_Regen_brake_torque_request"
  Signal Specification/1 -> Bus Creator/1  "BrkCtrl_Vehicle_speed"

== system CtrlStrct_VNT_Level1_TW/VNT_Level1_CAN_TW/HVAC_Ctrl/HVAC_Ctrl_VehCAN_Rx/HVAC_Ctrl_VehCAN_Receive_50ms ==
  VehCAN_Msg : Inport
  Bus Selector3 : BusSelector  OutputSignals=VM_Ctrl_VehCAN_Tx_0CFFD086
  HVAC_Ctrl_VehCAN Unpack : canmsglib/CAN Unpack  CANdbFile=HEV_CANDB.dbc  MsgList=Gateway_VehCAN_Tx_2  MsgName=Gateway_VehCAN_Tx_2  MsgIDType=Extended (29-bit identifier)  MsgIdentifier=218087813  MsgLength=8  SignalInfo=EngCtrl_Engine_speed_G$0$16$1$2$1$0$1.250000e-01$0$0$8192$#HEV_IdleStopCtrl_preparation_r_G$24$1$1$2$1$0$1$0$0$1$#HEV_IdleStopCtrl_request_G$25$1$1$2$1$0$1$0$0$1$#HEV_IdleStopCtrl_status_G$26$1$1$2$1$0$1$0$0$1$#TmCtrl_Gear_position_G$16$8$1$2$1$0$1$0$0$5$#  NSignals=5  IDPort=off  TimestampPort=off  ErrorPort=off  RemotePort=off  LengthPort=off  StatusPort=off  StartBits=str2num('[int32(0);int32(24);int32(25);int32(26);int32(16)]')  SignalSizes=str2num('[int32(16);int32(1);int32(1);int32(1);int32(8)]')  ByteOrders=str2num('[int32(1);int32(1);int32(1);int32(1);int32(1)]')  DataTypes=str2num('[int32(2);int32(2);int32(2);int32(2);int32(2)]')  MultiplexTypes=str2num('[int32(1);int32(1);int32(1);int32(1);int32(1)]')  MultiplexValues=str2num('[double(0);double(0);double(0);double(0);double(0)]')  Factors=str2num('[double(1.250000e-01);double(1);double(1);double(1);double(1)]')  Offsets=str2num('[double(0);double(0);double(0);double(0);double(0)]')  Minimums=str2num('[double(0);double(0);double(0);double(0);double(0)]')  Maximums=str2num('[double(8192);double(1);double(1);double(1);double(5)]')  ApplyMinMax=off
      settings: AttributesFormatString=<CANdbFile = %<CANdbFile>>  SourceProductName=Simulink Real-Time  SourceProductBaseCode=XP  DataFormat=CANdb specified signals
  Signal Specification : SignalSpecification
  Signal Specification1 : SignalSpecification
  Signal Specification2 : SignalSpecification
  Terminator6 : Terminator
  Terminator8 : Terminator
  EngCtrl_Engine_speed : Outport
  HEVCtrl_IdleStop_preparation_request : Outport  Port=2
  HEVCtrl_IdleStop_status : Outport  Port=3
  wires:
  HVAC_Ctrl_VehCAN Unpack/4 -> Signal Specification2/1  "VehCAN_HEVCtrl_IdleStop_status"
  HVAC_Ctrl_VehCAN Unpack/5 -> Terminator8/1
  HVAC_Ctrl_VehCAN Unpack/2 -> Signal Specification/1  "VehCAN_HEVCtrl_IdleStop_preparation_request"
  HVAC_Ctrl_VehCAN Unpack/3 -> Terminator6/1
  HVAC_Ctrl_VehCAN Unpack/1 -> Signal Specification1/1  "VehCAN_EngCtrl_Engine_speed"
  VehCAN_Msg/1 -> Bus Selector3/1
  Signal Specification/1 -> HEVCtrl_IdleStop_preparation_request/1  "HEVCtrl_IdleStop_preparation_request"
  Signal Specification1/1 -> EngCtrl_Engine_speed/1  "EngCtrl_Engine_speed"
  Signal Specification2/1 -> HEVCtrl_IdleStop_status/1  "HEVCtrl_IdleStop_status"
  Bus Selector3/1 -> HVAC_Ctrl_VehCAN Unpack/1  "<VM_Ctrl_VehCAN_Tx_0CFFD086>"
